simulink model "HW1_Mealy"  (R2017a)
settings: Solver=FixedStepDiscrete  StartTime=0.0  StopTime=inf  FixedStep=0.0001  RelTol=1e-3  EnableMultiTasking=on
settings Model: Creator=avise  LastModifiedBy=avise
settings SolverCC: AutoInsertRateTranBlk=on
settings DataIOCC: LimitDataPoints=on
settings OptimizationCC: LifeSpan=inf
settings DebuggingCC: AllowSymbolicDim=off  SFUnexpectedBacktrackingDiag=warning  SFNoUnconditionalDefaultTransitionDiag=warning  SFExecutionAtInitializationDiag=none
settings GRTTargetCC: TargetLangStandard=C89/C90 (ANSI)  GeneratePreprocessorConditionals=Disable all
settings ConfigComp: CovMetricSettings=dw  CovHtmlReporting=on  CovSaveCumulativeToWorkspaceVar=on  CovSaveSingleToWorkspaceVar=on  CovShowResultsExplorer=off  CovExternalEMLEnable=off  CovSFcnEnable=off

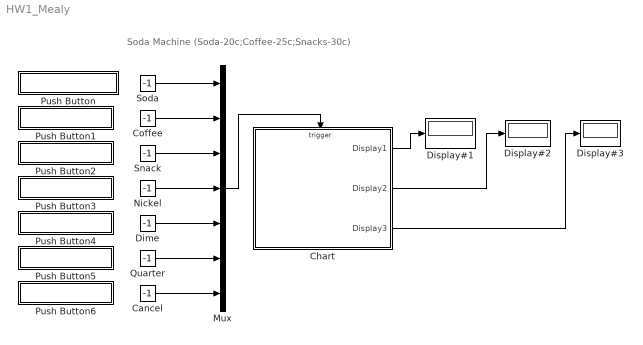
== system HW1_Mealy ==
  note: Soda Machine
      | (Soda-20c;Coffee-25c;Snacks-30c)
  Cancel : Constant  Value=-1
  Chart : Stateflow chart  TreatAsAtomicUnit=on
  Coffee : Constant  Value=-1
  Dime : Constant  Value=-1
  Display#1 : Display
  Display#2 : Display
  Display#3 : Display
  Mux : Mux  Inputs=7
  Nickel : Constant  Value=-1
  Push Button : Subsystem  DialogController=hmiCreateDDGDialog  IsWebBlock=on  mask(MWDashboardBlock){webBlockId=664f21db-061d-45c4-a5ed-301e6e3db717, webBlockType=pushbutton, ShowInLibBrwoser=on, ShowInitialText=on, HMISrcModelName=HW1_Mealy}
      mask prompts: webBlockId "WebBlock Id"; webBlockType "WebBlock Type"; HMISrcModelName "Source Model"
      mask help: SimulinkHMI:dialogs:PushButtonDialogDesc
      mask Help: helpview([docroot '/mapfiles/simulink.map'], 'hmi_push_button')
      mask Display:
      | model = bdroot(gcb);
      | if strcmp(get_param(model,'BlockDiagramType'), 'library')
      |     image([(matlabroot) '/toolbox/simulink/hmi/icons/PushButton.png']);
      | end
  Push Button1 : Subsystem  DialogController=hmiCreateDDGDialog  IsWebBlock=on  mask(MWDashboardBlock){webBlockId=369ec6e0-de46-472e-8dd1-8918505b40b8, webBlockType=pushbutton, ShowInLibBrwoser=on, ShowInitialText=on, HMISrcModelName=HW1_Mealy}
      mask prompts: webBlockId "WebBlock Id"; webBlockType "WebBlock Type"; HMISrcModelName "Source Model"
      mask help: SimulinkHMI:dialogs:PushButtonDialogDesc
      mask Help: helpview([docroot '/mapfiles/simulink.map'], 'hmi_push_button')
      mask Display:
      | model = bdroot(gcb);
      | if strcmp(get_param(model,'BlockDiagramType'), 'library')
      |     image([(matlabroot) '/toolbox/simulink/hmi/icons/PushButton.png']);
      | end
  Push Button2 : Subsystem  DialogController=hmiCreateDDGDialog  IsWebBlock=on  mask(MWDashboardBlock){webBlockId=437ecff1-f85d-43e6-a183-e5cb8b815949, webBlockType=pushbutton, ShowInLibBrwoser=on, ShowInitialText=on, HMISrcModelName=HW1_Mealy}
      mask prompts: webBlockId "WebBlock Id"; webBlockType "WebBlock Type"; HMISrcModelName "Source Model"
      mask help: SimulinkHMI:dialogs:PushButtonDialogDesc
      mask Help: helpview([docroot '/mapfiles/simulink.map'], 'hmi_push_button')
      mask Display:
      | model = bdroot(gcb);
      | if strcmp(get_param(model,'BlockDiagramType'), 'library')
      |     image([(matlabroot) '/toolbox/simulink/hmi/icons/PushButton.png']);
      | end
  Push Button3 : Subsystem  DialogController=hmiCreateDDGDialog  IsWebBlock=on  mask(MWDashboardBlock){webBlockId=f2e822cd-a8a7-4ab8-9e8e-7b39c5c413d8, webBlockType=pushbutton, ShowInLibBrwoser=on, ShowInitialText=on, HMISrcModelName=HW1_Mealy}
      mask prompts: webBlockId "WebBlock Id"; webBlockType "WebBlock Type"; HMISrcModelName "Source Model"
      mask help: SimulinkHMI:dialogs:PushButtonDialogDesc
      mask Help: helpview([docroot '/mapfiles/simulink.map'], 'hmi_push_button')
      mask Display:
      | model = bdroot(gcb);
      | if strcmp(get_param(model,'BlockDiagramType'), 'library')
      |     image([(matlabroot) '/toolbox/simulink/hmi/icons/PushButton.png']);
      | end
  Push Button4 : Subsystem  DialogController=hmiCreateDDGDialog  IsWebBlock=on  mask(MWDashboardBlock){webBlockId=f0c8a644-454f-4bf4-a778-a88d9125c533, webBlockType=pushbutton, ShowInLibBrwoser=on, ShowInitialText=on, HMISrcModelName=HW1_Mealy}
      mask prompts: webBlockId "WebBlock Id"; webBlockType "WebBlock Type"; HMISrcModelName "Source Model"
      mask help: SimulinkHMI:dialogs:PushButtonDialogDesc
      mask Help: helpview([docroot '/mapfiles/simulink.map'], 'hmi_push_button')
      mask Display:
      | model = bdroot(gcb);
      | if strcmp(get_param(model,'BlockDiagramType'), 'library')
      |     image([(matlabroot) '/toolbox/simulink/hmi/icons/PushButton.png']);
      | end
  Push Button5 : Subsystem  DialogController=hmiCreateDDGDialog  IsWebBlock=on  mask(MWDashboardBlock){webBlockId=21d649ba-39b7-4048-9903-c8ade3fb44d4, webBlockType=pushbutton, ShowInLibBrwoser=on, ShowInitialText=on, HMISrcModelName=HW1_Mealy}
      mask prompts: webBlockId "WebBlock Id"; webBlockType "WebBlock Type"; HMISrcModelName "Source Model"
      mask help: SimulinkHMI:dialogs:PushButtonDialogDesc
      mask Help: helpview([docroot '/mapfiles/simulink.map'], 'hmi_push_button')
      mask Display:
      | model = bdroot(gcb);
      | if strcmp(get_param(model,'BlockDiagramType'), 'library')
      |     image([(matlabroot) '/toolbox/simulink/hmi/icons/PushButton.png']);
      | end
  Push Button6 : Subsystem  DialogController=hmiCreateDDGDialog  IsWebBlock=on  mask(MWDashboardBlock){webBlockId=33373d40-ddda-4141-b1fc-f71dcaba8225, webBlockType=pushbutton, ShowInLibBrwoser=on, ShowInitialText=on, HMISrcModelName=HW1_Mealy}
      mask prompts: webBlockId "WebBlock Id"; webBlockType "WebBlock Type"; HMISrcModelName "Source Model"
      mask help: SimulinkHMI:dialogs:PushButtonDialogDesc
      mask Help: helpview([docroot '/mapfiles/simulink.map'], 'hmi_push_button')
      mask Display:
      | model = bdroot(gcb);
      | if strcmp(get_param(model,'BlockDiagramType'), 'library')
      |     image([(matlabroot) '/toolbox/simulink/hmi/icons/PushButton.png']);
      | end
  Quarter : Constant  Value=-1
  Snack : Constant  Value=-1
  Soda : Constant  Value=-1
  wires:
  Chart/1(Display1) -> Display#1/1
  Chart/2(Display2) -> Display#2/1
  Chart/3(Display3) -> Display#3/1
  Cancel/1 -> Mux/7
  Quarter/1 -> Mux/6
  Dime/1 -> Mux/5
  Nickel/1 -> Mux/4
  Snack/1 -> Mux/3
  Coffee/1 -> Mux/2
  Soda/1 -> Mux/1
  Mux/1 -> Chart/Trigger

== system HW1_Mealy/Push Button ==

== system HW1_Mealy/Push Button1 ==

== system HW1_Mealy/Push Button2 ==

== system HW1_Mealy/Push Button3 ==

== system HW1_Mealy/Push Button4 ==

== system HW1_Mealy/Push Button5 ==

== system HW1_Mealy/Push Button6 ==

== stateflow chart HW1_Mealy/Chart ==
  state Soda
    %20c
  state Wait
  state ReleaseorReset
    en:Reset
  state Error
  state Coffee
    %25c
  state Error1
  state Snack
    %30c
  state Error2
  (default) -> Wait
  Error -> (junction 34) [order 1] : Nickel{Display1=1;}
  Soda -> (junction 34) [order 1] : Nickel
  (junction 34) -> ReleaseorReset [order 1] : [Display2+5>=20]{Display2=Display2+5;Display3=Display2-20;}
  (junction 34) -> Soda [order 2] : [Display2+5<20]{Display2=Display2+5}
  Error -> (junction 45) [order 2] : Dime{Display1=1;}
  Wait -> Soda [order 5] : Soda{Display1=1;
      | Display3=-1;}
  Soda -> (junction 45) [order 2] : Dime
  (junction 45) -> ReleaseorReset [order 2] : [Display2+10>=20]{Display2=Display2+10;Display3=Display2-20;}
  (junction 45) -> Soda [order 1] : [Display2+10<20]{Display2=Display2+10;}
  Wait -> Coffee [order 6] : Coffee{Display1=2;
      | Display3=-1;}
  Wait -> Snack [order 7] : Snack{Display1=3;
      | Display3=-1;}
  Soda -> Error [order 5] : Coffee|Snack{Display1=9;}
  Soda -> (junction 49) [order 3] : Quarter
  (junction 49) -> ReleaseorReset : {Display2=Display2+25;Display3=Display2-20;}
  Error -> (junction 49) [order 3] : Quarter{Display1=1;}
  ReleaseorReset -> Wait : Reset{Display1=0;
      | Display2=0;}
  Soda -> ReleaseorReset [order 4] : Cancel{Display3=Display2;}
  Wait -> Wait [order 1] : Nickel{Display3=5;}
  Wait -> Wait [order 2] : Dime{Display3=10;}
  Wait -> Wait [order 3] : Quarter{Display3=25;}
  Wait -> Wait [order 4] : Cancel
  Error1 -> (junction 78) [order 2] : Nickel{Display1=2;}
  Error1 -> (junction 79) [order 1] : Dime{Display1=2;}
  Coffee -> (junction 78) [order 2] : Nickel
  (junction 78) -> ReleaseorReset [order 1] : [Display2+5>=25]{Display2=Display2+5;Display3=Display2-25;}
  (junction 78) -> Coffee [order 2] : [Display2+5<25]{Display2=Display2+5;}
  Coffee -> (junction 79) [order 1] : Dime
  (junction 79) -> ReleaseorReset [order 1] : [Display2+10>=25]{Display2=Display2+10;Display3=Display2-25;}
  (junction 79) -> Coffee [order 2] : [Display2+10<25]{Display2=Display2+10;}
  Coffee -> (junction 71) [order 3] : Quarter
  (junction 71) -> ReleaseorReset : {Display2=Display2+25;Display3=Display2-25;}
  Error1 -> (junction 71) [order 3] : Quarter{Display1=2;}
  Coffee -> ReleaseorReset [order 4] : Cancel{Display3=Display2;}
  Coffee -> Error1 [order 5] : Soda|Snack{Display1=9;}
  Error2 -> (junction 93) [order 2] : Nickel{Display1=3;}
  Snack -> (junction 93) [order 3] : Nickel
  (junction 93) -> ReleaseorReset [order 1] : [Display2+5>=30]{Display2=Display2+5;Display3=Display2-30;}
  (junction 93) -> Snack [order 2] : [Display2+5<30]{Display2=Display2+5;}
  Error2 -> (junction 95) [order 1] : Dime{Display1=3;}
  Snack -> (junction 95) [order 2] : Dime
  (junction 95) -> ReleaseorReset [order 1] : [Display2+10>=30]{Display2=Display2+10;Display3=Display2-30;}
  (junction 95) -> Snack [order 2] : [Display2+10<30]{Display2=Display2+10;}
  Snack -> (junction 94) [order 5] : Quarter
  (junction 94) -> ReleaseorReset [order 1] : [Display2+25>=30]{Display2=Display2+25;Display3=Display2-30;}
  Error2 -> (junction 94) [order 3] : Quarter{Display1=3;}
  (junction 94) -> Snack [order 2] : [Display2+25<30]{Display2=Display2+25;}
  Snack -> ReleaseorReset [order 1] : Cancel{Display3=Display2;}
  Snack -> Error2 [order 4] : Soda|Coffee{Display1=9;}
  data: Display1 output =0; Display2 output =0; Display3 output =-1
  events: Soda input EITHER_EDGE_EVENT; Coffee input EITHER_EDGE_EVENT; Snack input EITHER_EDGE_EVENT; Nickel input RISING_EDGE_EVENT; Dime input RISING_EDGE_EVENT; Quarter input RISING_EDGE_EVENT; Cancel input EITHER_EDGE_EVENT; Reset local FUNCTION_CALL_EVENT
